simulink model "SynchBuckSLX"  (R2016a)
settings: Solver=FixedStepDiscrete  StartTime=0.0  StopTime=10e-3  FixedStep=SampleTime  RelTol=1e-3
values from neighbouring files (symbols this model uses):
  Dbot = 19    [SynchBuckM.m]
  DelayBot = 50    [SynchBuckM.m]
  DelayTop = 0    [SynchBuckM.m]
  Dtop = 19    [SynchBuckM.m]
  fsw = 20e3    (= 20000)    [SynchBuckM.m]
  SampleTime = 1e-8    (= 1e-08)    [SynchBuckM.m]
  Vdc = 175    [SynchBuckM.m]
  VpulseMax = 6    [SynchBuckM.m]
  VpulseMin = -1    [SynchBuckM.m]
libraries: fl_lib x14, nesl_utility x12, elec_lib x5, simulink x3, pe_lib x2
settings Model: Creator=ugurm  LastModifiedBy=Furkan
settings OptimizationCC: EfficientMapNaN2IntZero=off
settings HardwareCC: TargetBitPerPointer=64  TargetLongLongMode=on  TargetIntDivRoundTo=Zero  TargetEndianess=LittleEndian  TargetWordSize=64  TargetHWDeviceType=MATLAB Host  ProdEqTarget=off
settings CodeAppCC: MaxIdLength=128
settings GRTTargetCC: GeneratePreprocessorConditionals=Use local settings  CombineOutputUpdateFcns=off  GRTInterface=on

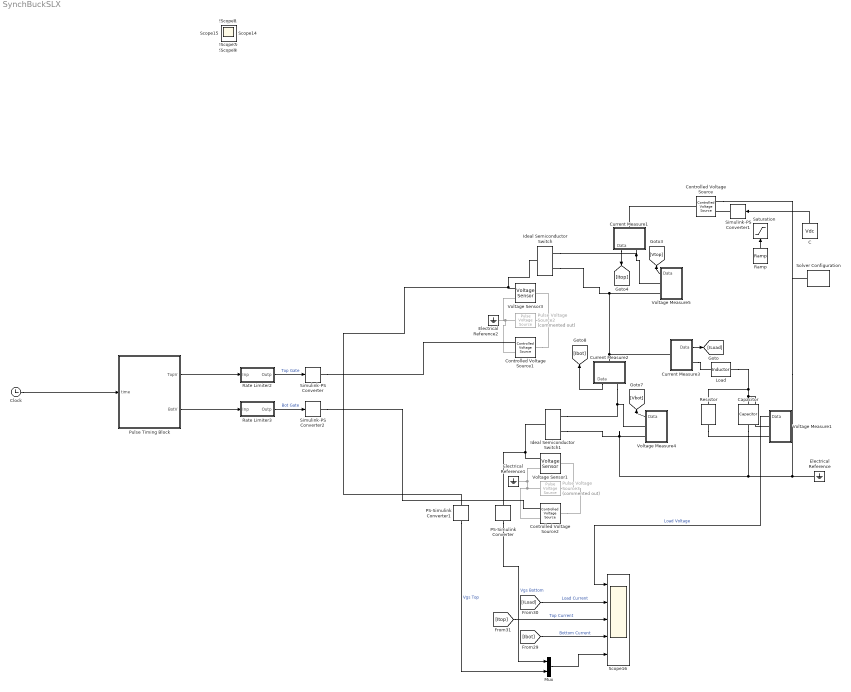
== system SynchBuckSLX ==
  "C " : Constant  Value=Vdc
  Capacitor : elec_lib/Passive Devices/Capacitor  enable_table=0  c=Cload F  Cvec=[ 1e-5 1e-6 ] F  Vvec=[ 0 10 ] V  CV_table_symmetry=1  C_tol=5  enable_C_tol=0  tol_distribution=1  nSigma=4  r=1e-6 Ohm  g=0 1/Ohm  initV=0 V  enable_operating_limits=0  operating_limit_action=2  max_working_voltage_range=[ -25 25 ] V  power_rating=1 W  enable_faults=0  fault_action=1  Cscale_faulted=100  R_faulted=0.001 Ohm  G_faulted=0 1/Ohm  tau_fault=0.001 s  enable_temporal_fault=0  t_fault=1 s  enable_behavioral_fault=0  max_permissible_voltage_range=[ -100 100 ] V  t_fail_on_voltage=1 s
  Clock : Clock
  Controlled Voltage Source : fl_lib/Electrical/Electrical Sources/Controlled Voltage Source
  Controlled Voltage Source1 : fl_lib/Electrical/Electrical Sources/Controlled Voltage Source
  Controlled Voltage Source2 : fl_lib/Electrical/Electrical Sources/Controlled Voltage Source
  Current Measure1 : Subsystem
  Current Measure2 : Subsystem
  Current Measure3 : Subsystem
  Electrical Reference : fl_lib/Electrical/Electrical Elements/Electrical Reference
  Electrical Reference1 : fl_lib/Electrical/Electrical Elements/Electrical Reference
  Electrical Reference2 : fl_lib/Electrical/Electrical Elements/Electrical Reference
  Ideal Semiconductor Switch : pe_lib/Semiconductors/Fundamental Components/Ideal Semiconductor Switch  Ron=0.001 Ohm  Goff=1e-6 1/Ohm  Vth=0.5 V  diode_param=2  diode_Vf=0.8 V  diode_Ron=0.001 Ohm  diode_Goff=1e-5 1/Ohm  diode_C=5e-8 F  diode_iRM=-235 A  diode_iF=300 A  diode_idot=-50 A/us  diode_trr_param=1  diode_trr_factor=3  diode_trr=15 us  diode_Qrr=1.5e+3 s*uA
  Ideal Semiconductor Switch1 : pe_lib/Semiconductors/Fundamental Components/Ideal Semiconductor Switch  Ron=0.001 Ohm  Goff=1e-6 1/Ohm  Vth=0.5 V  diode_param=2  diode_Vf=0.8 V  diode_Ron=0.001 Ohm  diode_Goff=1e-5 1/Ohm  diode_C=5e-8 F  diode_iRM=-235 A  diode_iF=300 A  diode_idot=-50 A/us  diode_trr_param=1  diode_trr_factor=3  diode_trr=15 us  diode_Qrr=1.5e+3 s*uA
  Load : elec_lib/Passive Devices/Inductor  l=Lload H  L_tol=20  enable_L_tol=0  tol_distribution=1  nSigma=4  r=0 Ohm  g=1e-9 1/Ohm  initI=InitialCurrent A  enable_operating_limits=0  operating_limit_action=2  max_working_current=1 A  power_rating=1 W  enable_faults=0  fault_action=1  lambdaPercent=50  k_faulted=0.9999 Ohm  turnsShort=0  openCct=0  groundShort=0  groundShortG=0 1/Ohm  tau_fault=0.001 s  enable_temporal_fault=0  t_fault=1 s  enable_behavioral_fault=0  max_permissible_voltage=100 V  n_fail_on_voltage=1  max_permissible_current=1 A  t_fail_on_current=1 s
  Mux : Mux  Inputs=2
  PS-Simulink Converter : nesl_utility/PS-Simulink Converter  PhysicalDomain=network_engine_domain  SubClassName=ps_output  LeftPortType=input  RightPortType=output  PseudoPeriodic=off  Frequencies=[]  Unit=1  AffineConversion=off
  PS-Simulink Converter1 : nesl_utility/PS-Simulink Converter  PhysicalDomain=network_engine_domain  SubClassName=ps_output  LeftPortType=input  RightPortType=output  PseudoPeriodic=off  Frequencies=[]  Unit=1  AffineConversion=off
  Pulse Timing Block : MATLAB Function  TreatAsAtomicUnit=on  SystemSampleTime=SampleTime
  Pulse Voltage Source2 : elec_lib/Additional Components/SPICE-Compatible Components/Sources/Pulse Voltage Source  Commented=on  V1=VpulseMin V  V2=VpulseMax V  TD=DelayTop/(100*fsw) s  TR=1e-9 s  TF=1e-9 s  PW=Dtop/(100*fsw) s  PER=1/fsw s
  Pulse Voltage Source3 : elec_lib/Additional Components/SPICE-Compatible Components/Sources/Pulse Voltage Source  Commented=on  V1=VpulseMin V  V2=VpulseMax V  TD=DelayBot/(100*fsw) s  TR=1e-9 s  TF=1e-9 s  PW=Dbot/(100*fsw) s  PER=1/fsw s
  Ramp : simulink/Sources/Ramp  slope=Vdc/9e-6  start=0  X0=0
  Rate Limiter2 : Subsystem
  Rate Limiter3 : Subsystem
  Resistor : elec_lib/Passive Devices/Resistor  R=30 Ohm  R_tol=5  enable_R_tol=0  tol_distribution=1  nSigma=4  enable_operating_limits=0  operating_limit_action=2  max_working_voltage=100 V  power_rating=1 W  enable_faults=0  fault_action=1  R_faulted=Inf Ohm  enable_temporal_fault=0  t_fault=1 s  enable_behavioral_fault=0  max_permissible_current=1 A  t_fail_on_current=1 s  noise_mode=0  sample_time=0.001 s  repeatability=1  auto_seed=4013553621  user_seed=0  Tdevice=25 degC  alpha=0.00393 1/K  Tmeas=25 degC  thermal_mass=100 J/K  initial_temperature=25 degC  power_derating_T1=70 degC  power_derating_T2=155 degC  operating_temperature_range_vec=[ -50 150 ] degC
  Saturation : Saturate  UpperLimit=Vdc  LowerLimit=0
  Scope16 : Scope  NumInputPorts=5
  Simulink-PS Converter : nesl_utility/Simulink-PS Converter  PhysicalDomain=network_engine_domain  SubClassName=ps_input  LeftPortType=input  RightPortType=output  PseudoPeriodic=off  Frequencies=[]  NoiseDistribution=none  NoiseParameters=[]  Unit=1  AffineConversion=off  InputFiltering=off  SimscapeFilterOrder=1  InputFilterTimeConstant=0.001  UdotUserProvided=1
  Simulink-PS Converter1 : nesl_utility/Simulink-PS Converter  PhysicalDomain=network_engine_domain  SubClassName=ps_input  LeftPortType=input  RightPortType=output  PseudoPeriodic=off  Frequencies=[]  NoiseDistribution=none  NoiseParameters=[]  Unit=1  AffineConversion=off  InputFiltering=off  SimscapeFilterOrder=1  InputFilterTimeConstant=0.001  UdotUserProvided=1
  Simulink-PS Converter2 : nesl_utility/Simulink-PS Converter  PhysicalDomain=network_engine_domain  SubClassName=ps_input  LeftPortType=input  RightPortType=output  PseudoPeriodic=off  Frequencies=[]  NoiseDistribution=none  NoiseParameters=[]  Unit=1  AffineConversion=off  InputFiltering=off  SimscapeFilterOrder=1  InputFilterTimeConstant=0.001  UdotUserProvided=1
  Solver Configuration : nesl_utility/Solver Configuration  PhysicalDomain=network_engine_domain  SubClassName=solver  LeftPortType=input  RightPortType=generic  Accelerate=off  Tones=[]  Harmonics=[]  SimulateNoise=off  Profile=off  UseLocalSampling=off  EnableSwitchedLinearOptims=on  FrequencyDomain=off  UseCCode=off  RelTol=0.001  AbsTol=1e-06  MinStep=1e-09  ToWorkspace=off  RevertToSquareIcSolve=off  NumHomotopyIterations=100  PhasorMode=off  PhasorModeNumHarmonics=1  OverrideAbsTol=off  DoDC=off  ResidualTolerance=1e-09  UseLocalSolver=on  LocalSolverChoice=NE_BACKWARD_EULER_ADVANCER  LocalSolverSampleTime=SampleTime  DoFixedCost=on  MaxNonlinIter=3  MaxModeIter=2  LinearAlgebra=Sparse  DelaysMemoryBudget=1024  AutomaticFiltering=on  FilteringTimeConstant=0.001
  Voltage Measure1 : Subsystem
  Voltage Measure4 : Subsystem
  Voltage Measure5 : Subsystem
  Voltage Sensor1 : fl_lib/Electrical/Electrical Sensors/Voltage Sensor
  Voltage Sensor3 : fl_lib/Electrical/Electrical Sensors/Voltage Sensor
  Scope{7..11,13..15} (8 alike) : Scope
  wires:
  Current Measure3/1(Data) -> [ILoad]
  Voltage Measure4/1(Data) -> [Vbot]
  Voltage Measure5/1(Data) -> [Vtop]
  Current Measure1/1(Data) -> [Itop]
  Current Measure2/1(Data) -> [Ibot]
  [Ibot] -> Scope16/4  "Bottom Current"
  Ramp/1 -> Saturation/1
  [Itop] -> Scope16/3  "Top Current"
  [ILoad] -> Scope16/2  "Load Current"
  Voltage Measure1/1(Data) -> Scope16/1  "Load Voltage"
  Clock/1 -> Pulse Timing Block/1(time)
  Pulse Timing Block/2(BotV) -> Rate Limiter3/1(Inp)
  Pulse Timing Block/1(TopV) -> Rate Limiter2/1(Inp)
  Rate Limiter2/1(Outp) -> Simulink-PS Converter/1  "Top Gate"
  Rate Limiter3/1(Outp) -> Simulink-PS Converter2/1  "Bot Gate"
  Mux/1 -> Scope16/5
  PS-Simulink Converter/1 -> Mux/1  "Vgs Bottom"
  PS-Simulink Converter1/1 -> Mux/2  "Vgs Top"
  "C "/1 -> Simulink-PS Converter1/1
  connections:
  Current Measure1/RConn1 -- Ideal Semiconductor Switch/RConn1 -- Voltage Measure5/RConn1
  Current Measure2/RConn1 -- Ideal Semiconductor Switch1/RConn1 -- Voltage Measure4/RConn1
  Controlled Voltage Source/LConn1 -- Current Measure1/LConn1
  Controlled Voltage Source/RConn2 -- Solver Configuration/RConn1 -- Resistor/RConn1 -- Capacitor/RConn1 -- Voltage Measure1/RConn2 -- Ideal Semiconductor Switch1/RConn2 -- Voltage Measure4/RConn2 -- Electrical Reference/LConn1
  Current Measure2/LConn1 -- Ideal Semiconductor Switch/RConn2 -- Voltage Measure5/RConn2 -- Current Measure3/LConn1
  Current Measure3/RConn1 -- Load/LConn1
  Load/RConn1 -- Resistor/LConn1 -- Voltage Measure1/RConn1 -- Capacitor/LConn1
  Pulse Voltage Source2/RConn1 -- Controlled Voltage Source1/RConn2 -- Voltage Sensor3/RConn2 -- Electrical Reference2/LConn1
  Pulse Voltage Source2/LConn1 -- Controlled Voltage Source1/LConn1 -- Voltage Sensor3/LConn1
  Voltage Sensor3/RConn1 -- PS-Simulink Converter1/LConn1 -- Ideal Semiconductor Switch/LConn1
  Pulse Voltage Source3/LConn1 -- Controlled Voltage Source2/LConn1 -- Voltage Sensor1/LConn1
  Pulse Voltage Source3/RConn1 -- Controlled Voltage Source2/RConn2 -- Electrical Reference1/LConn1 -- Voltage Sensor1/RConn2
  Voltage Sensor1/RConn1 -- PS-Simulink Converter/LConn1 -- Ideal Semiconductor Switch1/LConn1
  Simulink-PS Converter1/RConn1 -- Controlled Voltage Source/RConn1
  Simulink-PS Converter/RConn1 -- Controlled Voltage Source1/RConn1
  Simulink-PS Converter2/RConn1 -- Controlled Voltage Source2/RConn1

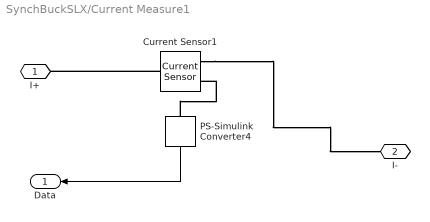
== system SynchBuckSLX/Current Measure1 ==
  Current Sensor1 : fl_lib/Electrical/Electrical Sensors/Current Sensor
  PS-Simulink Converter4 : nesl_utility/PS-Simulink Converter  PhysicalDomain=network_engine_domain  SubClassName=ps_output  LeftPortType=input  RightPortType=output  PseudoPeriodic=off  Frequencies=[]  Unit=1  AffineConversion=off
  I+ : PMIOPort  Port=1  Side=Left
  I- : PMIOPort  Port=2  Side=Right
  Data : Outport
  wires:
  PS-Simulink Converter4/1 -> Data/1
  connections:
  Current Sensor1/RConn2 -- I-/RConn1
  PS-Simulink Converter4/LConn1 -- Current Sensor1/RConn1
  Current Sensor1/LConn1 -- I+/RConn1

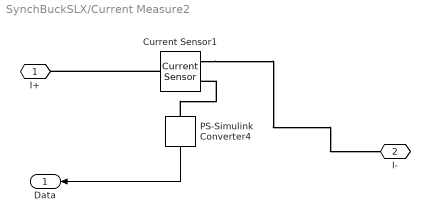
== system SynchBuckSLX/Current Measure2 ==
  Current Sensor1 : fl_lib/Electrical/Electrical Sensors/Current Sensor
  PS-Simulink Converter4 : nesl_utility/PS-Simulink Converter  PhysicalDomain=network_engine_domain  SubClassName=ps_output  LeftPortType=input  RightPortType=output  PseudoPeriodic=off  Frequencies=[]  Unit=1  AffineConversion=off
  I+ : PMIOPort  Port=1  Side=Left
  I- : PMIOPort  Port=2  Side=Right
  Data : Outport
  wires:
  PS-Simulink Converter4/1 -> Data/1
  connections:
  Current Sensor1/RConn2 -- I-/RConn1
  PS-Simulink Converter4/LConn1 -- Current Sensor1/RConn1
  Current Sensor1/LConn1 -- I+/RConn1

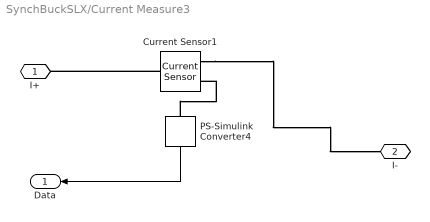
== system SynchBuckSLX/Current Measure3 ==
  Current Sensor1 : fl_lib/Electrical/Electrical Sensors/Current Sensor
  PS-Simulink Converter4 : nesl_utility/PS-Simulink Converter  PhysicalDomain=network_engine_domain  SubClassName=ps_output  LeftPortType=input  RightPortType=output  PseudoPeriodic=off  Frequencies=[]  Unit=1  AffineConversion=off
  I+ : PMIOPort  Port=1  Side=Left
  I- : PMIOPort  Port=2  Side=Right
  Data : Outport
  wires:
  PS-Simulink Converter4/1 -> Data/1
  connections:
  Current Sensor1/LConn1 -- I+/RConn1
  PS-Simulink Converter4/LConn1 -- Current Sensor1/RConn1
  Current Sensor1/RConn2 -- I-/RConn1

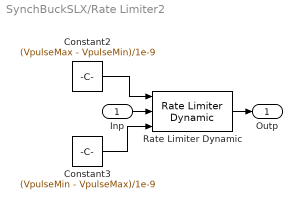
== system SynchBuckSLX/Rate Limiter2 ==
  Inp : Inport
  Constant2 : Constant  Value=(VpulseMax - VpulseMin)/1e-9
  Constant3 : Constant  Value=(VpulseMin - VpulseMax)/1e-9
  Rate Limiter Dynamic : simulink/Discontinuities/Rate Limiter Dynamic
  Outp : Outport
  wires:
  Constant3/1 -> Rate Limiter Dynamic/3
  Constant2/1 -> Rate Limiter Dynamic/1
  Inp/1 -> Rate Limiter Dynamic/2
  Rate Limiter Dynamic/1 -> Outp/1

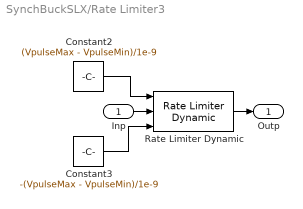
== system SynchBuckSLX/Rate Limiter3 ==
  Inp : Inport
  Constant2 : Constant  Value=(VpulseMax - VpulseMin)/1e-9
  Constant3 : Constant  Value=-(VpulseMax - VpulseMin)/1e-9
  Rate Limiter Dynamic : simulink/Discontinuities/Rate Limiter Dynamic
  Outp : Outport
  wires:
  Rate Limiter Dynamic/1 -> Outp/1
  Inp/1 -> Rate Limiter Dynamic/2
  Constant2/1 -> Rate Limiter Dynamic/1
  Constant3/1 -> Rate Limiter Dynamic/3

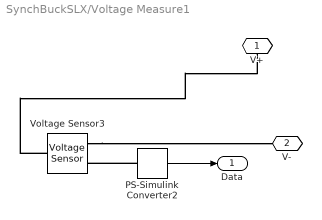
== system SynchBuckSLX/Voltage Measure1 ==
  PS-Simulink Converter2 : nesl_utility/PS-Simulink Converter  PhysicalDomain=network_engine_domain  SubClassName=ps_output  LeftPortType=input  RightPortType=output  PseudoPeriodic=off  Frequencies=[]  Unit=1  AffineConversion=off
  Voltage Sensor3 : fl_lib/Electrical/Electrical Sensors/Voltage Sensor
  V+ : PMIOPort  Port=1  Side=Right
  V- : PMIOPort  Port=2  Side=Right
  Data : Outport
  wires:
  PS-Simulink Converter2/1 -> Data/1
  connections:
  PS-Simulink Converter2/LConn1 -- Voltage Sensor3/RConn1
  Voltage Sensor3/RConn2 -- V-/RConn1
  Voltage Sensor3/LConn1 -- V+/RConn1

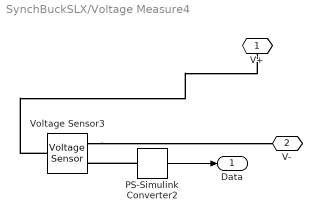
== system SynchBuckSLX/Voltage Measure4 ==
  PS-Simulink Converter2 : nesl_utility/PS-Simulink Converter  PhysicalDomain=network_engine_domain  SubClassName=ps_output  LeftPortType=input  RightPortType=output  PseudoPeriodic=off  Frequencies=[]  Unit=1  AffineConversion=off
  Voltage Sensor3 : fl_lib/Electrical/Electrical Sensors/Voltage Sensor
  V+ : PMIOPort  Port=1  Side=Right
  V- : PMIOPort  Port=2  Side=Right
  Data : Outport
  wires:
  PS-Simulink Converter2/1 -> Data/1
  connections:
  Voltage Sensor3/LConn1 -- V+/RConn1
  Voltage Sensor3/RConn2 -- V-/RConn1
  PS-Simulink Converter2/LConn1 -- Voltage Sensor3/RConn1

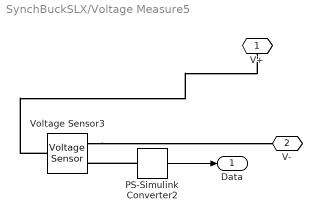
== system SynchBuckSLX/Voltage Measure5 ==
  PS-Simulink Converter2 : nesl_utility/PS-Simulink Converter  PhysicalDomain=network_engine_domain  SubClassName=ps_output  LeftPortType=input  RightPortType=output  PseudoPeriodic=off  Frequencies=[]  Unit=1  AffineConversion=off
  Voltage Sensor3 : fl_lib/Electrical/Electrical Sensors/Voltage Sensor
  V+ : PMIOPort  Port=1  Side=Right
  V- : PMIOPort  Port=2  Side=Right
  Data : Outport
  wires:
  PS-Simulink Converter2/1 -> Data/1
  connections:
  PS-Simulink Converter2/LConn1 -- Voltage Sensor3/RConn1
  Voltage Sensor3/RConn2 -- V-/RConn1
  Voltage Sensor3/LConn1 -- V+/RConn1

== matlab function SynchBuckSLX/Pulse Timing Block ==
  data: TopV output; BotV output; time input
function [TopV,BotV]= fcn(time)
fsw = 20e3;
Vdc = 175;
VpulseMax = 6;
VpulseMin = 0;
Dtop = 49; % duty cycle of top
Dbot = 49; % duty cycle of bot
DelayTop = 50;
DelayBot = 50;
LoadCurrent = 15;
Rload = (Vdc*Dtop/100)/LoadCurrent;
Lload = 1e-3;
% Cload = 100e-6;
CurrRipple = (LoadCurrent*Rload)*(1-0.01*Dtop)/(fsw*Lload);
% VoltRipple = CurrRipple/(8*fsw*Cload);
ReqTime = 5e-3; %Lload*(LoadCurrent)/(Vdc - (Vdc*(Dtop/2/100)-10)); %20 to compensate increase in output voltage
Dtop = time*49/ReqTime;
if Dtop > 49
    Dtop = 49;
end
Dbot = 100 - Dtop - 2;
PseudoTime = time - ReqTime;
% if PseudoTime >= 0 
    while PseudoTime > 1/fsw
        PseudoTime = PseudoTime - 1/fsw;
    end
    if (PseudoTime >= 0 && PseudoTime < (Dbot/100)/fsw) %bottom on top off dead time öncesi
        TopV = VpulseMin;
        BotV = VpulseMax;
   elseif (PseudoTime >= ((Dbot/100)/fsw) && PseudoTime < ((1-DelayBot/100)/fsw))%bottom off oldu top off zaten dead time
        TopV = VpulseMin;
        BotV = VpulseMin;
    elseif PseudoTime >= ((DelayTop/100)/fsw) && PseudoTime < ((0.5 + Dtop/100)/fsw) %% top on bottom off dead time öncesi
        TopV = VpulseMax;
        BotV = VpulseMin;
    else
        TopV = VpulseMin;
        BotV = VpulseMin;
    end
    
% else
%     if time >= (ReqTime - ((100 - Dtop - DelayTop)/100)/fsw)
%     TopV = VpulseMin;
%     BotV = VpulseMin;
%     else
%     TopV = VpulseMax;
%     BotV = VpulseMin; 
%     end
% end
